simulink model "IEEE_14_Final"  (R2024a)
settings: Solver=FixedStepDiscrete  StartTime=0  StopTime=0.20000000000000001  FixedStep=0.00016666666666666666  RelTol=1e-4  AbsTol=1e-6  EnableMultiTasking=on
undefined symbols (not defined in the file or in its folder): D11, Delta
libraries: spsThreePhasePISectionLineLib x21, spsThreePhaseVIMeasurementLib x17, spsThreePhaseSeriesRLCLoadLib x11, spsGroundLib x9, spsThreePhaseTransformerTwoWindingsLib x6, spsThreePhaseFaultLib x4, spsSynchronousMachinepuStandardLib x3, spsThreePhaseParallelRLCBranchLib x3, sps_lib x1
settings Model: Creator=Bharath  LastModifiedBy=Shakkya Gamage
settings SolverCC: AutoScaleAbsTol=off  MaxConsecutiveMinStep=auto  ZeroCrossControl=DisableAll  AlgebraicLoopSolver=TrustRegion
settings DataIOCC: SaveFormat=Array  SignalLoggingSaveFormat=ModelDataLogs
settings OptimizationCC: ExpressionDepthLimit=2147483647  LifeSpan=inf
settings DebuggingCC: AlgebraicLoopMsg=none  UnderspecifiedInitializationDetection=Classic  MergeDetectMultiDrivingBlocksExec=none  FcnCallInpInsideContextMsg=warning  UnconnectedInputMsg=warning  UnconnectedLineMsg=warning  StateNameClashWarn=warning  SFUnexpectedBacktrackingDiag=warning  SFNoUnconditionalDefaultTransitionDiag=warning  SFExecutionAtInitializationDiag=none  ArithmeticOperatorsInVariantConditions=warning
settings HardwareCC: ProdBitPerPointer=32  ProdBitPerSizeT=32  ProdBitPerPtrDiffT=32  ProdLargestAtomicFloat=None  ProdIntDivRoundTo=Undefined  ProdEndianess=Unspecified  ProdWordSize=32  ProdHWDeviceType=32-bit Generic
settings ModelReferenceCC: PropagateSignalLabelsOutOfModel=off
settings SFSimCC: SimUseLocalCustomCode=off  CustomCodeUndefinedFunction=UseInterfaceOnly
settings RTWCC: RTWUseLocalCustomCode=off  GPUComputeCapability=3.5
settings CodeAppCC: StateflowObjectComments=on
settings GRTTargetCC: TargetLangStandard=C89/C90 (ANSI)  CombineOutputUpdateFcns=off  GRTInterface=on
settings ConfigComp: CovMetricSettings=dw  CovSaveCumulativeToWorkspaceVar=on  CovSaveSingleToWorkspaceVar=on  CovExternalEMLEnable=off
settings SimscapeCC: SimscapeNormalizeSystem=off

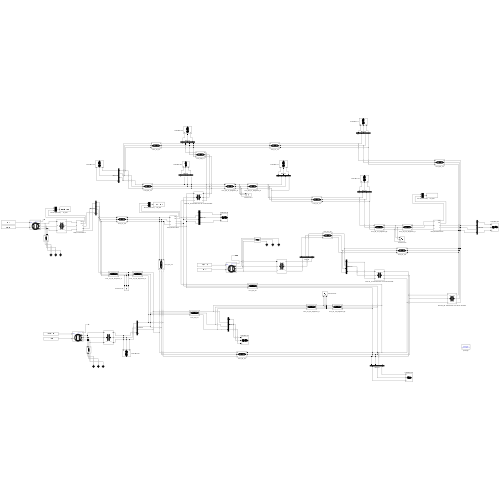
[thumbnail: Simulink's stored preview of the top-level diagram]
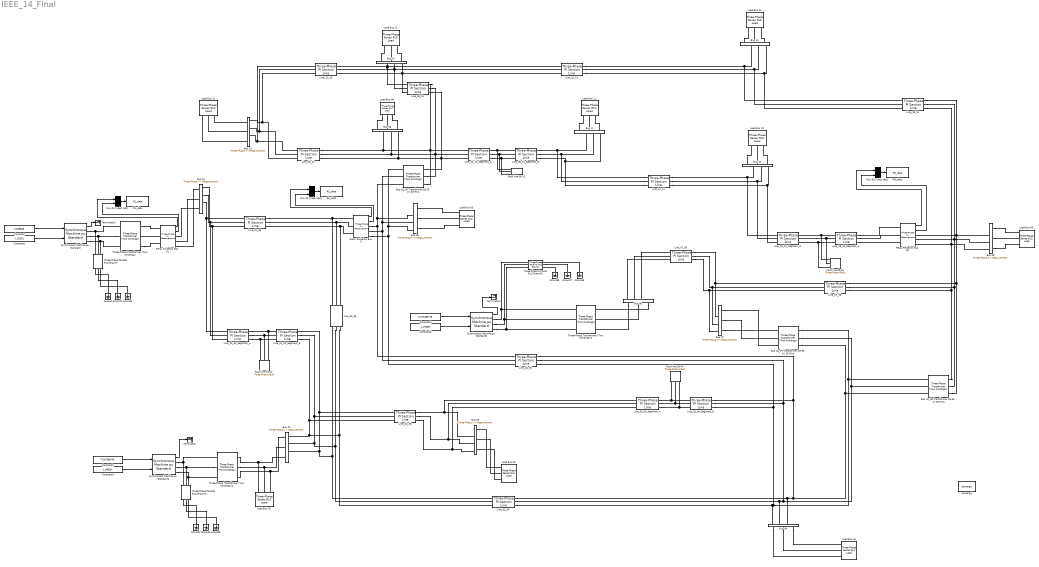
== system IEEE_14_Final ==
  Bus 01 : spsThreePhaseVIMeasurementLib/Three-Phase V-I Measurement  VoltageMeasurement=phase-to-ground  SetLabelV=off  LabelV=Vabc  Vpu=off  VpuLL=off  CurrentMeasurement=no  SetLabelI=off  LabelI=Iabc  Ipu=off  Pbase=31500000  Vbase=33000  OutputType=Complex  PhasorSimulation=off  PSBequivalent=0
  Bus 02 : spsThreePhaseVIMeasurementLib/Three-Phase V-I Measurement  VoltageMeasurement=phase-to-ground  SetLabelV=off  LabelV=Vabc  Vpu=off  VpuLL=off  CurrentMeasurement=no  SetLabelI=off  LabelI=Iabc  Ipu=off  Pbase=31500000  Vbase=33000  OutputType=Complex  PhasorSimulation=off  PSBequivalent=0
  Bus 03 : spsThreePhaseVIMeasurementLib/Three-Phase V-I Measurement  VoltageMeasurement=phase-to-ground  SetLabelV=off  LabelV=Vabc  Vpu=off  VpuLL=off  CurrentMeasurement=no  SetLabelI=off  LabelI=Iabc  Ipu=off  Pbase=31500000  Vbase=33000  OutputType=Complex  PhasorSimulation=off  PSBequivalent=0
  Bus 04 : spsThreePhaseVIMeasurementLib/Three-Phase V-I Measurement  VoltageMeasurement=phase-to-ground  SetLabelV=off  LabelV=Vabc  Vpu=off  VpuLL=off  CurrentMeasurement=no  SetLabelI=off  LabelI=Iabc  Ipu=off  Pbase=31500000  Vbase=33000  OutputType=Complex  PhasorSimulation=off  PSBequivalent=0
  Bus 04_07 Transformer 33-33 kV 50 MVA : spsThreePhaseTransformerTwoWindingsLib/Three-Phase Transformer (Two Windings)  Winding1Connection=Yg  Winding2Connection=Yg  CoreType=Three single-phase transformers  SetSaturation=off  Hysteresis=off  DataFile='hysteresis'  SetInitialFlux=off  Measurements=None  UNITS=pu  NominalPower=[50000000, 50]  Winding1=[33000 0.005 0.05]  Winding2=[33000 0.005 0.05]  Rm=500  Lm=500  L0=0.5  Saturation=[ 0,0 ; 0.0024,1.2 ; 1.0,1.52 ]  InitialFluxes=[ 0.8 , -0.8 , 0.7 ]  BreakLoop=off  DiscreteSolver=Trapezoidal iterative  DataType=off  TransfoNumber=1
  Bus 04_09 Transformer 33-33 kV 50 MVA : spsThreePhaseTransformerTwoWindingsLib/Three-Phase Transformer (Two Windings)  Winding1Connection=Yg  Winding2Connection=Yg  CoreType=Three single-phase transformers  SetSaturation=off  Hysteresis=off  DataFile='hysteresis'  SetInitialFlux=off  Measurements=None  UNITS=pu  NominalPower=[50000000, 50]  Winding1=[33000 0.005 0.14]  Winding2=[33000 0.005 0.14]  Rm=500  Lm=500  L0=0.5  Saturation=[ 0,0 ; 0.0024,1.2 ; 1.0,1.52 ]  InitialFluxes=[ 0.8 , -0.8 , 0.7 ]  BreakLoop=off  DiscreteSolver=Trapezoidal iterative  DataType=off  TransfoNumber=1
  Bus 05 : spsThreePhaseVIMeasurementLib/Three-Phase V-I Measurement  VoltageMeasurement=phase-to-ground  SetLabelV=off  LabelV=Vabc  Vpu=off  VpuLL=off  CurrentMeasurement=no  SetLabelI=off  LabelI=Iabc  Ipu=off  Pbase=31500000  Vbase=33000  OutputType=Complex  PhasorSimulation=off  PSBequivalent=0
  Bus 05_06 Transformer 33-33 kV 50 MVA : spsThreePhaseTransformerTwoWindingsLib/Three-Phase Transformer (Two Windings)  Winding1Connection=Yg  Winding2Connection=Yg  CoreType=Three single-phase transformers  SetSaturation=off  Hysteresis=off  DataFile='hysteresis'  SetInitialFlux=off  Measurements=None  UNITS=pu  NominalPower=[50000000, 50]  Winding1=[33000 0.005 0.063]  Winding2=[33000 0.005 0.063]  Rm=500  Lm=500  L0=0.5  Saturation=[ 0,0 ; 0.0024,1.2 ; 1.0,1.52 ]  InitialFluxes=[ 0.8 , -0.8 , 0.7 ]  BreakLoop=off  DiscreteSolver=Trapezoidal iterative  DataType=off  TransfoNumber=1
  Bus 06 : spsThreePhaseVIMeasurementLib/Three-Phase V-I Measurement  VoltageMeasurement=phase-to-ground  SetLabelV=off  LabelV=Vabc  Vpu=off  VpuLL=off  CurrentMeasurement=no  SetLabelI=off  LabelI=Iabc  Ipu=off  Pbase=31500000  Vbase=33000  OutputType=Complex  PhasorSimulation=off  PSBequivalent=0
  Bus 07 : spsThreePhaseVIMeasurementLib/Three-Phase V-I Measurement  VoltageMeasurement=phase-to-ground  SetLabelV=off  LabelV=Vabc  Vpu=off  VpuLL=off  CurrentMeasurement=no  SetLabelI=off  LabelI=Iabc  Ipu=off  Pbase=31500000  Vbase=33000  OutputType=Complex  PhasorSimulation=off  PSBequivalent=0
  Bus 08 : spsThreePhaseVIMeasurementLib/Three-Phase V-I Measurement  VoltageMeasurement=phase-to-ground  SetLabelV=off  LabelV=Vabc  Vpu=off  VpuLL=off  CurrentMeasurement=no  SetLabelI=off  LabelI=Iabc  Ipu=off  Pbase=31500000  Vbase=33000  OutputType=Complex  PhasorSimulation=off  PSBequivalent=0
  Bus 09 : spsThreePhaseVIMeasurementLib/Three-Phase V-I Measurement  VoltageMeasurement=phase-to-ground  SetLabelV=off  LabelV=Vabc  Vpu=off  VpuLL=off  CurrentMeasurement=no  SetLabelI=off  LabelI=Iabc  Ipu=off  Pbase=31500000  Vbase=33000  OutputType=Complex  PhasorSimulation=off  PSBequivalent=0
  Bus {10..14} (5 alike) : spsThreePhaseVIMeasurementLib/Three-Phase V-I Measurement  VoltageMeasurement=phase-to-ground  SetLabelV=off  LabelV=Vabc  Vpu=off  VpuLL=off  CurrentMeasurement=no  SetLabelI=off  LabelI=Iabc  Ipu=off  Pbase=31500000  Vbase=33000  OutputType=Complex  PhasorSimulation=off  PSBequivalent=0
  Constant : Constant  Value=0.205826
  Constant1 : Constant  Value=1.02301
  Constant2 : Constant  Value=7.51429e-06
  Constant3 : Constant  Value=1.09059
  Constant4 : Constant  Value=5.27348e-06
  Constant5 : Constant  Value=1.07589
  Fault line 01-02 : spsThreePhaseFaultLib/Three-Phase Fault  InitialStates=0  FaultA=off  FaultB=off  FaultC=off  GroundFault=off  SwitchTimes=[100 100.1]  External=off  SwitchStatus=NaN  FaultResistance=0.01  GroundResistance=0.001  SnubberResistance=1e6  SnubberCapacitance=inf  Measurements=None
  Fault line 03-04 : spsThreePhaseFaultLib/Three-Phase Fault  InitialStates=0  FaultA=off  FaultB=off  FaultC=off  GroundFault=off  SwitchTimes=[100 100.1]  External=off  SwitchStatus=NaN  FaultResistance=0.01  GroundResistance=0.001  SnubberResistance=1e6  SnubberCapacitance=inf  Measurements=None
  Fault line 06-11 : spsThreePhaseFaultLib/Three-Phase Fault  InitialStates=0  FaultA=off  FaultB=off  FaultC=off  GroundFault=off  SwitchTimes=[100 100.1]  External=off  SwitchStatus=NaN  FaultResistance=0.01  GroundResistance=0.001  SnubberResistance=1e6  SnubberCapacitance=inf  Measurements=None
  Fault line 09-10 : spsThreePhaseFaultLib/Three-Phase Fault  InitialStates=0  FaultA=on  FaultB=on  FaultC=on  GroundFault=off  SwitchTimes=[0.089158 0.128934]  External=off  SwitchStatus=NaN  FaultResistance=0.01  GroundResistance=0.001  SnubberResistance=1e6  SnubberCapacitance=inf  Measurements=None
  Ground{,1..8} (9 alike) : spsGroundLib/Ground  LConnTagsString=a
  Line_01_02_Segment_A : spsThreePhasePISectionLineLib/Three-Phase PI Section Line  LConnTagsString=A|B|C  RConnTagsString=A|B|C  Length=10  Frequency=50  Resistances=[0.16 0.48]  Inductances=[0.0012 0.0036]  Capacitances=[1e-08 6e-09]
  Line_01_02_Segment_B : spsThreePhasePISectionLineLib/Three-Phase PI Section Line  LConnTagsString=A|B|C  RConnTagsString=A|B|C  Length=10  Frequency=50  Resistances=[0.16 0.48]  Inductances=[0.0012 0.0036]  Capacitances=[1e-08 6e-09]
  Line_01_05 : spsThreePhasePISectionLineLib/Three-Phase PI Section Line  LConnTagsString=A|B|C  RConnTagsString=A|B|C  Length=15  Frequency=50  Resistances=[0.16 0.48]  Inductances=[0.0012 0.0036]  Capacitances=[1e-08 6e-09]
  Line_02_03 : spsThreePhasePISectionLineLib/Three-Phase PI Section Line  LConnTagsString=A|B|C  RConnTagsString=A|B|C  Length=12  Frequency=50  Resistances=[0.16 0.48]  Inductances=[0.0012 0.0036]  Capacitances=[1e-08 6e-09]
  Line_02_04 : spsThreePhasePISectionLineLib/Three-Phase PI Section Line  LConnTagsString=A|B|C  RConnTagsString=A|B|C  Length=10  Frequency=50  Resistances=[0.16 0.48]  Inductances=[0.0012 0.0036]  Capacitances=[1e-08 6e-09]
  Line_02_05 : spsThreePhasePISectionLineLib/Three-Phase PI Section Line  LConnTagsString=A|B|C  RConnTagsString=A|B|C  Length=8  Frequency=50  Resistances=[0.16 0.48]  Inductances=[0.0012 0.0036]  Capacitances=[1e-08 6e-09]
  Line_03_04_Segment_A : spsThreePhasePISectionLineLib/Three-Phase PI Section Line  LConnTagsString=A|B|C  RConnTagsString=A|B|C  Length=9  Frequency=50  Resistances=[0.16 0.48]  Inductances=[0.0012 0.0036]  Capacitances=[1e-08 6e-09]
  Line_03_04_Segment_B : spsThreePhasePISectionLineLib/Three-Phase PI Section Line  LConnTagsString=A|B|C  RConnTagsString=A|B|C  Length=9  Frequency=50  Resistances=[0.16 0.48]  Inductances=[0.0012 0.0036]  Capacitances=[1e-08 6e-09]
  Line_04_05 : spsThreePhasePISectionLineLib/Three-Phase PI Section Line  LConnTagsString=A|B|C  RConnTagsString=A|B|C  Length=7  Frequency=50  Resistances=[0.16 0.48]  Inductances=[0.0012 0.0036]  Capacitances=[1e-08 6e-09]
  Line_06_11_Segment_A : spsThreePhasePISectionLineLib/Three-Phase PI Section Line  LConnTagsString=A|B|C  RConnTagsString=A|B|C  Length=4  Frequency=50  Resistances=[0.16 0.48]  Inductances=[0.0012 0.0036]  Capacitances=[1e-08 6e-09]
  Line_06_11_Segment_B : spsThreePhasePISectionLineLib/Three-Phase PI Section Line  LConnTagsString=A|B|C  RConnTagsString=A|B|C  Length=4  Frequency=50  Resistances=[0.16 0.48]  Inductances=[0.0012 0.0036]  Capacitances=[1e-08 6e-09]
  Line_06_12 : spsThreePhasePISectionLineLib/Three-Phase PI Section Line  LConnTagsString=A|B|C  RConnTagsString=A|B|C  Length=12  Frequency=50  Resistances=[0.16 0.48]  Inductances=[0.0012 0.0036]  Capacitances=[1e-08 6e-09]
  Line_06_13 : spsThreePhasePISectionLineLib/Three-Phase PI Section Line  LConnTagsString=A|B|C  RConnTagsString=A|B|C  Length=15  Frequency=50  Resistances=[0.16 0.48]  Inductances=[0.0012 0.0036]  Capacitances=[1e-08 6e-09]
  Line_07_08 : spsThreePhasePISectionLineLib/Three-Phase PI Section Line  LConnTagsString=A|B|C  RConnTagsString=A|B|C  Length=5  Frequency=50  Resistances=[0.16 0.48]  Inductances=[0.0012 0.0036]  Capacitances=[1e-08 6e-09]
  Line_07_09 : spsThreePhasePISectionLineLib/Three-Phase PI Section Line  LConnTagsString=A|B|C  RConnTagsString=A|B|C  Length=8  Frequency=50  Resistances=[0.16 0.48]  Inductances=[0.0012 0.0036]  Capacitances=[1e-08 6e-09]
  Line_09_10_Segment_A : spsThreePhasePISectionLineLib/Three-Phase PI Section Line  LConnTagsString=A|B|C  RConnTagsString=A|B|C  Length=1.6926369239615902  Frequency=50  Resistances=[0.16 0.48]  Inductances=[0.0012 0.0036]  Capacitances=[1e-08 6e-09]
  Line_09_10_Segment_B : spsThreePhasePISectionLineLib/Three-Phase PI Section Line  LConnTagsString=A|B|C  RConnTagsString=A|B|C  Length=8.3073630760384098  Frequency=50  Resistances=[0.16 0.48]  Inductances=[0.0012 0.0036]  Capacitances=[1e-08 6e-09]
  Line_09_14 : spsThreePhasePISectionLineLib/Three-Phase PI Section Line  LConnTagsString=A|B|C  RConnTagsString=A|B|C  Length=14  Frequency=50  Resistances=[0.16 0.48]  Inductances=[0.0012 0.0036]  Capacitances=[1e-08 6e-09]
  Line_10_11 : spsThreePhasePISectionLineLib/Three-Phase PI Section Line  LConnTagsString=A|B|C  RConnTagsString=A|B|C  Length=6  Frequency=50  Resistances=[0.16 0.48]  Inductances=[0.0012 0.0036]  Capacitances=[1e-08 6e-09]
  Line_12_13 : spsThreePhasePISectionLineLib/Three-Phase PI Section Line  LConnTagsString=A|B|C  RConnTagsString=A|B|C  Length=5  Frequency=50  Resistances=[0.16 0.48]  Inductances=[0.0012 0.0036]  Capacitances=[1e-08 6e-09]
  Line_13_14 : spsThreePhasePISectionLineLib/Three-Phase PI Section Line  LConnTagsString=A|B|C  RConnTagsString=A|B|C  Length=7  Frequency=50  Resistances=[0.16 0.48]  Inductances=[0.0012 0.0036]  Capacitances=[1e-08 6e-09]
  Load Bus 02 : spsThreePhaseSeriesRLCLoadLib/Three-Phase Series RLC Load  LConnTagsString=A|B|C  Configuration=Y (grounded)  NominalVoltage=33000  Vabc=[1e3 1e3 1e3]  Vabcp=[1e3 1e3 1e3]  NominalFrequency=50  UnbalancedPower=off  ActivePower=500000  InductivePower=100000  CapacitivePower=0  Pabc=[10e3 9e3 11e3]  QLabc=[100 90 110]  QCabc=[100 90 110]  Pabcp=[10e3 9e3 11e3]  QLabcp=[100 90 110]  QCabcp=[100 90 110]  Measurements=None  LoadType=constant PQ
  Load Bus 03 : spsThreePhaseSeriesRLCLoadLib/Three-Phase Series RLC Load  LConnTagsString=A|B|C  Configuration=Y (grounded)  NominalVoltage=33000  Vabc=[1e3 1e3 1e3]  Vabcp=[1e3 1e3 1e3]  NominalFrequency=50  UnbalancedPower=off  ActivePower=500000  InductivePower=100000  CapacitivePower=0  Pabc=[10e3 9e3 11e3]  QLabc=[100 90 110]  QCabc=[100 90 110]  Pabcp=[10e3 9e3 11e3]  QLabcp=[100 90 110]  QCabcp=[100 90 110]  Measurements=None  LoadType=constant PQ
  Load Bus 04 : spsThreePhaseSeriesRLCLoadLib/Three-Phase Series RLC Load  LConnTagsString=A|B|C  Configuration=Y (grounded)  NominalVoltage=33000  Vabc=[1e3 1e3 1e3]  Vabcp=[1e3 1e3 1e3]  NominalFrequency=50  UnbalancedPower=off  ActivePower=3000000  InductivePower=0  CapacitivePower=0  Pabc=[10e3 9e3 11e3]  QLabc=[100 90 110]  QCabc=[100 90 110]  Pabcp=[10e3 9e3 11e3]  QLabcp=[100 90 110]  QCabcp=[100 90 110]  Measurements=None  LoadType=constant PQ
  Load Bus 05 : spsThreePhaseSeriesRLCLoadLib/Three-Phase Series RLC Load  LConnTagsString=A|B|C  Configuration=Y (grounded)  NominalVoltage=33000  Vabc=[1e3 1e3 1e3]  Vabcp=[1e3 1e3 1e3]  NominalFrequency=50  UnbalancedPower=off  ActivePower=500000  InductivePower=100000  CapacitivePower=0  Pabc=[10e3 9e3 11e3]  QLabc=[100 90 110]  QCabc=[100 90 110]  Pabcp=[10e3 9e3 11e3]  QLabcp=[100 90 110]  QCabcp=[100 90 110]  Measurements=None  LoadType=constant PQ
  Load Bus 06 : spsThreePhaseSeriesRLCLoadLib/Three-Phase Series RLC Load  LConnTagsString=A|B|C  Configuration=Y (grounded)  NominalVoltage=33000  Vabc=[1e3 1e3 1e3]  Vabcp=[1e3 1e3 1e3]  NominalFrequency=50  UnbalancedPower=off  ActivePower=500000  InductivePower=100000  CapacitivePower=0  Pabc=[10e3 9e3 11e3]  QLabc=[100 90 110]  QCabc=[100 90 110]  Pabcp=[10e3 9e3 11e3]  QLabcp=[100 90 110]  QCabcp=[100 90 110]  Measurements=None  LoadType=constant PQ
  Load Bus 09 : spsThreePhaseSeriesRLCLoadLib/Three-Phase Series RLC Load  LConnTagsString=A|B|C  Configuration=Y (grounded)  NominalVoltage=33000  Vabc=[1e3 1e3 1e3]  Vabcp=[1e3 1e3 1e3]  NominalFrequency=50  UnbalancedPower=off  ActivePower=1800000  InductivePower=1000000  CapacitivePower=0  Pabc=[10e3 9e3 11e3]  QLabc=[100 90 110]  QCabc=[100 90 110]  Pabcp=[10e3 9e3 11e3]  QLabcp=[100 90 110]  QCabcp=[100 90 110]  Measurements=None  LoadType=constant PQ
  Load Bus 10 : spsThreePhaseSeriesRLCLoadLib/Three-Phase Series RLC Load  LConnTagsString=A|B|C  Configuration=Y (grounded)  NominalVoltage=33000  Vabc=[1e3 1e3 1e3]  Vabcp=[1e3 1e3 1e3]  NominalFrequency=50  UnbalancedPower=off  ActivePower=600000  InductivePower=400000  CapacitivePower=0  Pabc=[10e3 9e3 11e3]  QLabc=[100 90 110]  QCabc=[100 90 110]  Pabcp=[10e3 9e3 11e3]  QLabcp=[100 90 110]  QCabcp=[100 90 110]  Measurements=None  LoadType=constant PQ
  Load Bus 11 : spsThreePhaseSeriesRLCLoadLib/Three-Phase Series RLC Load  LConnTagsString=A|B|C  Configuration=Y (grounded)  NominalVoltage=33000  Vabc=[1e3 1e3 1e3]  Vabcp=[1e3 1e3 1e3]  NominalFrequency=50  UnbalancedPower=off  ActivePower=200000  InductivePower=100000  CapacitivePower=0  Pabc=[10e3 9e3 11e3]  QLabc=[100 90 110]  QCabc=[100 90 110]  Pabcp=[10e3 9e3 11e3]  QLabcp=[100 90 110]  QCabcp=[100 90 110]  Measurements=None  LoadType=constant PQ
  Load Bus 12 : spsThreePhaseSeriesRLCLoadLib/Three-Phase Series RLC Load  LConnTagsString=A|B|C  Configuration=Y (grounded)  NominalVoltage=33000  Vabc=[1e3 1e3 1e3]  Vabcp=[1e3 1e3 1e3]  NominalFrequency=50  UnbalancedPower=off  ActivePower=400000  InductivePower=100000  CapacitivePower=0  Pabc=[10e3 9e3 11e3]  QLabc=[100 90 110]  QCabc=[100 90 110]  Pabcp=[10e3 9e3 11e3]  QLabcp=[100 90 110]  QCabcp=[100 90 110]  Measurements=None  LoadType=constant PQ
  Load Bus 13 : spsThreePhaseSeriesRLCLoadLib/Three-Phase Series RLC Load  LConnTagsString=A|B|C  Configuration=Y (grounded)  NominalVoltage=33000  Vabc=[1e3 1e3 1e3]  Vabcp=[1e3 1e3 1e3]  NominalFrequency=50  UnbalancedPower=off  ActivePower=800000  InductivePower=400000  CapacitivePower=0  Pabc=[10e3 9e3 11e3]  QLabc=[100 90 110]  QCabc=[100 90 110]  Pabcp=[10e3 9e3 11e3]  QLabcp=[100 90 110]  QCabcp=[100 90 110]  Measurements=None  LoadType=constant PQ
  Load Bus 14 : spsThreePhaseSeriesRLCLoadLib/Three-Phase Series RLC Load  LConnTagsString=A|B|C  Configuration=Y (grounded)  NominalVoltage=33000  Vabc=[1e3 1e3 1e3]  Vabcp=[1e3 1e3 1e3]  NominalFrequency=50  UnbalancedPower=off  ActivePower=900000  InductivePower=300000  CapacitivePower=0  Pabc=[10e3 9e3 11e3]  QLabc=[100 90 110]  QCabc=[100 90 110]  Pabcp=[10e3 9e3 11e3]  QLabcp=[100 90 110]  QCabcp=[100 90 110]  Measurements=None  LoadType=constant PQ
  Mux R1 [Vabc Iabc] : Mux  Inputs=2
  Mux R5 [Vabc Iabc] : Mux  Inputs=2
  Mux R9 [Vabc Iabc] : Mux  Inputs=2
  R1_data : ToWorkspace  VariableName=R1_data  SampleTime=-1
  R5_data : ToWorkspace  VariableName=R5_data  SampleTime=-1
  R9_data : ToWorkspace  VariableName=R9_data  SampleTime=-1
  Relay R1 below Bus 01 : spsThreePhaseVIMeasurementLib/Three-Phase V-I Measurement  VoltageMeasurement=phase-to-ground  SetLabelV=off  LabelV=Vabc  Vpu=off  VpuLL=off  CurrentMeasurement=yes  SetLabelI=off  LabelI=Iabc  Ipu=off  Pbase=31500000  Vbase=33000  OutputType=Complex  PhasorSimulation=off  PSBequivalent=0
  Relay R5 below Bus 5 : spsThreePhaseVIMeasurementLib/Three-Phase V-I Measurement  VoltageMeasurement=phase-to-ground  SetLabelV=off  LabelV=Vabc  Vpu=off  VpuLL=off  CurrentMeasurement=yes  SetLabelI=off  LabelI=Iabc  Ipu=off  Pbase=31500000  Vbase=33000  OutputType=Complex  PhasorSimulation=off  PSBequivalent=0
  Relay R9 below Bus 09 : spsThreePhaseVIMeasurementLib/Three-Phase V-I Measurement  VoltageMeasurement=phase-to-ground  SetLabelV=off  LabelV=Vabc  Vpu=off  VpuLL=off  CurrentMeasurement=yes  SetLabelI=off  LabelI=Iabc  Ipu=off  Pbase=31500000  Vbase=33000  OutputType=Complex  PhasorSimulation=off  PSBequivalent=0
  Synchronous Machine pu Standard : spsSynchronousMachinepuStandardLib/Synchronous Machine pu Standard  PresetModel=No  MechanicalLoad=Mechanical power Pm  ShowDetailedParameters=on  RotorType=Round  Units=per unit standard parameters  MeasurementBus=off  NominalParameters=[50e6 11e3 50]  Reactances1=[1.81 0.30 0.23 1.76 0.65 0.25 0.15]  Reactances2=[2.24 0.17 0.12 1.02 0.13 0.08]  dAxisTimeConstants=Open-circuit  qAxisTimeConstants=Open-circuit  TimeConstants1="[ 4.4849  0.0681  0.1  ]"  TimeConstants2=[ 8.0, 0.03, 1.0, 0.07 ]  TimeConstants3="[  4.49  0.0681  0.0513  ]"  TimeConstants4=[ 8.0, 0.03, 0.3371, 0.0295 ]  TimeConstants5=[ 1.01, 0.053, 0.1 ]  TimeConstants6=[ 1.3201, 0.023, 1.0, 0.07 ]  TimeConstants7=[0.012 0.003 0.003]  TimeConstants8=[ 8.0 0.03 1.0 0.07 ]  StatorResistance=0.003  Mechanical=[3.5 0 1]  PolePairs=20  InitialConditions=[0 -69.219 0.20738 0.20738 0.20738 7.30633 -112.694 127.306 1.02301]  SetSaturation=off  Saturation=[0.6404,0.7127,0.8441,0.9214,0.9956,1.082,1.19,1.316,1.457;0.7,0.7698,0.8872,0.9466,0.9969,1.046,1.1,1.151,1.201]  LoadFlowParameters=[2 0 0 0 0]  TsPowergui=0  TsBlock=-1  IterativeModel=Trapezoidal non iterative  IterativeDiscreteModel=Trapezoidal robust  BusType=swing  Pref=0  Qref=0  Qmin=-inf  Qmax=inf  PLF=0  QLF=0
  Synchronous Machine pu Standard1 : spsSynchronousMachinepuStandardLib/Synchronous Machine pu Standard  PresetModel=No  MechanicalLoad=Mechanical power Pm  ShowDetailedParameters=on  RotorType=Round  Units=per unit standard parameters  MeasurementBus=off  NominalParameters=[50e6 11e3 50]  Reactances1=[1.81 0.30 0.23 1.76 0.65 0.25 0.15]  Reactances2=[2.24 0.17 0.12 1.02 0.13 0.08]  dAxisTimeConstants=Open-circuit  qAxisTimeConstants=Open-circuit  TimeConstants1="[ 4.4849  0.0681  0.1  ]"  TimeConstants2=[ 8.0, 0.03, 1.0, 0.07 ]  TimeConstants3="[  4.49  0.0681  0.0513  ]"  TimeConstants4=[ 8.0, 0.03, 0.3371, 0.0295 ]  TimeConstants5=[ 1.01, 0.053, 0.1 ]  TimeConstants6=[ 1.3201, 0.023, 1.0, 0.07 ]  TimeConstants7=[0.012 0.003 0.003]  TimeConstants8=[ 8.0 0.03 1.0 0.07 ]  StatorResistance=0.003  Mechanical=[3.5 0 1]  PolePairs=20  InitialConditions=[0 -93.0795 0.0500476 0.0500476 0.0500476 -93.0716 146.928 26.9284 1.09059]  SetSaturation=off  Saturation=[0.6404,0.7127,0.8441,0.9214,0.9956,1.082,1.19,1.316,1.457;0.7,0.7698,0.8872,0.9466,0.9969,1.046,1.1,1.151,1.201]  LoadFlowParameters=[1 0 0 0 0]  TsPowergui=0  TsBlock=-1  IterativeModel=Trapezoidal non iterative  IterativeDiscreteModel=Trapezoidal robust  BusType=swing  Pref=0  Qref=0  Qmin=-inf  Qmax=inf  PLF=0  QLF=0
  Synchronous Machine pu Standard2 : spsSynchronousMachinepuStandardLib/Synchronous Machine pu Standard  PresetModel=No  MechanicalLoad=Mechanical power Pm  ShowDetailedParameters=on  RotorType=Round  Units=per unit standard parameters  MeasurementBus=off  NominalParameters=[50e6 11e3 50]  Reactances1=[1.81 0.30 0.23 1.76 0.65 0.25 0.15]  Reactances2=[2.24 0.17 0.12 1.02 0.13 0.08]  dAxisTimeConstants=Open-circuit  qAxisTimeConstants=Open-circuit  TimeConstants1="[ 4.4849  0.0681  0.1  ]"  TimeConstants2=[ 8.0, 0.03, 1.0, 0.07 ]  TimeConstants3="[  4.49  0.0681  0.0513  ]"  TimeConstants4=[ 8.0, 0.03, 0.3371, 0.0295 ]  TimeConstants5=[ 1.01, 0.053, 0.1 ]  TimeConstants6=[ 1.3201, 0.023, 1.0, 0.07 ]  TimeConstants7=[0.012 0.003 0.003]  TimeConstants8=[ 8.0 0.03 1.0 0.07 ]  StatorResistance=0.003  Mechanical=[3.5 0 1]  PolePairs=20  InitialConditions=[0 -93.7473 0.0419264 0.0419264 0.0419264 -93.7406 146.259 26.2594 1.07589]  SetSaturation=off  Saturation=[0.6404,0.7127,0.8441,0.9214,0.9956,1.082,1.19,1.316,1.457;0.7,0.7698,0.8872,0.9466,0.9969,1.046,1.1,1.151,1.201]  LoadFlowParameters=[1 0 0 0 0]  TsPowergui=0  TsBlock=-1  IterativeModel=Trapezoidal non iterative  IterativeDiscreteModel=Trapezoidal robust  BusType=swing  Pref=0  Qref=0  Qmin=-inf  Qmax=inf  PLF=0  QLF=0
  Terminator : Terminator
  Terminator1 : Terminator
  Terminator2 : Terminator
  Three-Phase Parallel RLC Branch : spsThreePhaseParallelRLCBranchLib/Three-Phase Parallel RLC Branch  LConnTagsString=A|B|C  RConnTagsString=A|B|C  BranchType=R  Resistance=1e6  Inductance=1e-3  Capacitance=1e-6  Measurements=None
  Three-Phase Parallel RLC Branch1 : spsThreePhaseParallelRLCBranchLib/Three-Phase Parallel RLC Branch  LConnTagsString=A|B|C  RConnTagsString=A|B|C  BranchType=R  Resistance=1e6  Inductance=1e-3  Capacitance=1e-6  Measurements=None
  Three-Phase Parallel RLC Branch2 : spsThreePhaseParallelRLCBranchLib/Three-Phase Parallel RLC Branch  LConnTagsString=A|B|C  RConnTagsString=A|B|C  BranchType=R  Resistance=1e6  Inductance=1e-3  Capacitance=1e-6  Measurements=None
  Three-Phase Transformer (Two Windings) : spsThreePhaseTransformerTwoWindingsLib/Three-Phase Transformer (Two Windings)  Winding1Connection=Delta (D11)  Winding2Connection=Yg  CoreType=Three single-phase transformers  SetSaturation=off  Hysteresis=off  DataFile='hysteresis'  SetInitialFlux=off  Measurements=None  UNITS=pu  NominalPower=[ 50e6 , 50 ]  Winding1=[ 11e3 , 0.005 , 0.05 ]  Winding2=[ 33e3 , 0.005 , 0.05 ]  Rm=500  Lm=500  L0=0.5  Saturation=[ 0,0 ; 0.0024,1.2 ; 1.0,1.52 ]  InitialFluxes=[ 0.8 , -0.8 , 0.7 ]  BreakLoop=off  DiscreteSolver=Trapezoidal iterative  DataType=off  TransfoNumber=1
  Three-Phase Transformer (Two Windings)1 : spsThreePhaseTransformerTwoWindingsLib/Three-Phase Transformer (Two Windings)  Winding1Connection=Delta (D11)  Winding2Connection=Yg  CoreType=Three single-phase transformers  SetSaturation=off  Hysteresis=off  DataFile='hysteresis'  SetInitialFlux=off  Measurements=None  UNITS=pu  NominalPower=[ 50e6 , 50 ]  Winding1=[ 11e3 , 0.005 , 0.05 ]  Winding2=[ 33e3 , 0.005 , 0.05 ]  Rm=500  Lm=500  L0=0.5  Saturation=[ 0,0 ; 0.0024,1.2 ; 1.0,1.52 ]  InitialFluxes=[ 0.8 , -0.8 , 0.7 ]  BreakLoop=off  DiscreteSolver=Trapezoidal iterative  DataType=off  TransfoNumber=1
  Three-Phase Transformer (Two Windings)2 : spsThreePhaseTransformerTwoWindingsLib/Three-Phase Transformer (Two Windings)  Winding1Connection=Delta (D11)  Winding2Connection=Yg  CoreType=Three single-phase transformers  SetSaturation=off  Hysteresis=off  DataFile='hysteresis'  SetInitialFlux=off  Measurements=None  UNITS=pu  NominalPower=[ 50e6 , 50 ]  Winding1=[ 11e3 , 0.005 , 0.05 ]  Winding2=[ 33e3 , 0.005 , 0.05 ]  Rm=500  Lm=500  L0=0.5  Saturation=[ 0,0 ; 0.0024,1.2 ; 1.0,1.52 ]  InitialFluxes=[ 0.8 , -0.8 , 0.7 ]  BreakLoop=off  DiscreteSolver=Trapezoidal iterative  DataType=off  TransfoNumber=1
  powergui : sps_lib/powergui  Priority=1  SimulationMode=Discrete  SampleTime=1/6000  frequency=50  Iterations=50  frequencyindice=50  Pbase=31500000  ErrMax=1e-4  UnitsV=kV  UnitsW=MW  buscounter=0  FunctionMessages=off  echomessages=off  EnableUseOfTLC=off  CurrentSourceSwitches=on  DisableSnubberDevices=off  DisableRonSwitches=off  DisableVfSwitches=off  DisplayEquations=off  AutomaticDiscreteSolvers=off  SolverType=Tustin  Interpol=off  ExternalGateDelay=off  methode=off  Ts=100  x0status=blocks  SPID=off  SwTol=0  HookPort=off  NonlinearTolerance=1e-4  nMaxIteration=100  ContinueOnMaxIteration=off  RestoreLinks=warning  ResistiveCurrentMeasurement=off  Frange=[0:2:500]  Ylog=off  Xlog=on  ShowGrid=off  save=off  variable=ZData  structure=0  ZoomFFT=off  StartTime=0.0  cycles=1  DisplayStyle=1  fundamental=50  FreqAxis=off  MaxFrequency=3000  frequencyindicesteady=1  RmsSteady=1  display=off
  wires:
  Relay R1 below Bus 01/1 -> Mux R1 [Vabc Iabc]/1
  Relay R1 below Bus 01/2 -> Mux R1 [Vabc Iabc]/2
  Mux R1 [Vabc Iabc]/1 -> R1_data/1
  Mux R9 [Vabc Iabc]/1 -> R9_data/1
  Relay R9 below Bus 09/2 -> Mux R9 [Vabc Iabc]/2
  Relay R9 below Bus 09/1 -> Mux R9 [Vabc Iabc]/1
  Mux R5 [Vabc Iabc]/1 -> R5_data/1
  Relay R5 below Bus 5/2 -> Mux R5 [Vabc Iabc]/2
  Relay R5 below Bus 5/1 -> Mux R5 [Vabc Iabc]/1
  Constant1/1 -> Synchronous Machine pu Standard/2
  Constant/1 -> Synchronous Machine pu Standard/1
  Constant2/1 -> Synchronous Machine pu Standard1/1
  Constant3/1 -> Synchronous Machine pu Standard1/2
  Constant4/1 -> Synchronous Machine pu Standard2/1
  Constant5/1 -> Synchronous Machine pu Standard2/2
  Synchronous Machine pu Standard1/1 -> Terminator/1
  Synchronous Machine pu Standard/1 -> Terminator1/1
  Synchronous Machine pu Standard2/1 -> Terminator2/1
  connections:
  Bus 01/RConn1 -- Line_01_02_Segment_A/LConn1 -- Line_01_05/LConn1
  Line_01_05/RConn1 -- Relay R5 below Bus 5/LConn1 -- Line_02_05/RConn1
  Bus 08/RConn1 -- Line_07_08/RConn1
  Bus 01/RConn2 -- Line_01_05/LConn2 -- Line_01_02_Segment_A/LConn2
  Line_04_05/LConn2 -- Relay R5 below Bus 5/RConn2 -- Bus 05/RConn2 -- Bus 05_06 Transformer 33-33 kV 50 MVA/LConn2
  Bus 08/RConn2 -- Line_07_08/RConn2
  Bus 01/RConn3 -- Line_01_02_Segment_A/LConn3 -- Line_01_05/LConn3
  Line_04_05/LConn3 -- Relay R5 below Bus 5/RConn3 -- Bus 05/RConn3 -- Bus 05_06 Transformer 33-33 kV 50 MVA/LConn3
  Bus 08/RConn3 -- Line_07_08/RConn3
  Load Bus 03/LConn1 -- Bus 03/LConn1
  Load Bus 03/LConn2 -- Bus 03/LConn2
  Load Bus 03/LConn3 -- Bus 03/LConn3
  Bus 04/LConn1 -- Load Bus 04/LConn1
  Bus 04/LConn2 -- Load Bus 04/LConn2
  Bus 04/LConn3 -- Load Bus 04/LConn3
  Bus 05/LConn1 -- Load Bus 05/LConn1
  Bus 05/LConn2 -- Load Bus 05/LConn2
  Bus 05/LConn3 -- Load Bus 05/LConn3
  Load Bus 06/LConn1 -- Bus 06/LConn1
  Load Bus 06/LConn2 -- Bus 06/LConn2
  Load Bus 06/LConn3 -- Bus 06/LConn3
  Bus 09/LConn1 -- Load Bus 09/LConn1
  Bus 09/LConn2 -- Load Bus 09/LConn2
  Bus 09/LConn3 -- Load Bus 09/LConn3
  Bus 10/LConn1 -- Load Bus 10/LConn1
  Bus 10/LConn2 -- Load Bus 10/LConn2
  Bus 10/LConn3 -- Load Bus 10/LConn3
  Bus 11/LConn1 -- Load Bus 11/LConn1
  Bus 11/LConn2 -- Load Bus 11/LConn2
  Bus 11/LConn3 -- Load Bus 11/LConn3
  Bus 12/LConn1 -- Load Bus 12/LConn1
  Bus 12/LConn2 -- Load Bus 12/LConn2
  Bus 12/LConn3 -- Load Bus 12/LConn3
  Bus 13/LConn1 -- Load Bus 13/LConn1
  Bus 13/LConn2 -- Load Bus 13/LConn2
  Bus 13/LConn3 -- Load Bus 13/LConn3
  Bus 14/LConn1 -- Load Bus 14/LConn1
  Bus 14/LConn2 -- Load Bus 14/LConn2
  Bus 14/LConn3 -- Load Bus 14/LConn3
  Relay R1 below Bus 01/RConn1 -- Bus 01/LConn1
  Relay R1 below Bus 01/RConn2 -- Bus 01/LConn2
  Relay R1 below Bus 01/RConn3 -- Bus 01/LConn3
  Line_01_02_Segment_A/RConn1 -- Line_01_02_Segment_B/LConn1 -- Fault line 01-02/LConn1
  Line_01_02_Segment_A/RConn2 -- Fault line 01-02/LConn2 -- Line_01_02_Segment_B/LConn2
  Line_01_02_Segment_A/RConn3 -- Line_01_02_Segment_B/LConn3 -- Fault line 01-02/LConn3
  Line_03_04_Segment_A/RConn1 -- Line_03_04_Segment_B/LConn1 -- Fault line 03-04/LConn1
  Line_03_04_Segment_A/RConn2 -- Line_03_04_Segment_B/LConn2 -- Fault line 03-04/LConn2
  Line_03_04_Segment_A/RConn3 -- Line_03_04_Segment_B/LConn3 -- Fault line 03-04/LConn3
  Line_09_10_Segment_A/RConn1 -- Fault line 09-10/LConn1 -- Line_09_10_Segment_B/LConn1
  Line_09_10_Segment_A/RConn2 -- Fault line 09-10/LConn2 -- Line_09_10_Segment_B/LConn2
  Line_09_10_Segment_A/RConn3 -- Fault line 09-10/LConn3 -- Line_09_10_Segment_B/LConn3
  Line_01_02_Segment_B/RConn1 -- Line_02_04/LConn1 -- Line_02_05/LConn1 -- Bus 02/RConn1 -- Line_02_03/LConn1
  Line_01_02_Segment_B/RConn2 -- Line_02_05/LConn2 -- Line_02_04/LConn2 -- Bus 02/RConn2 -- Line_02_03/LConn2
  Line_01_02_Segment_B/RConn3 -- Line_02_04/LConn3 -- Line_02_05/LConn3 -- Bus 02/RConn3 -- Line_02_03/LConn3
  Line_02_03/RConn1 -- Line_03_04_Segment_A/LConn1 -- Bus 03/RConn1
  Line_02_03/RConn2 -- Line_03_04_Segment_A/LConn2 -- Bus 03/RConn2
  Line_02_03/RConn3 -- Line_03_04_Segment_A/LConn3 -- Bus 03/RConn3
  Line_06_13/LConn1 -- Bus 05_06 Transformer 33-33 kV 50 MVA/RConn1 -- Line_06_11_Segment_A/RConn1 -- Line_06_12/LConn1 -- Bus 06/RConn1
  Line_06_12/LConn2 -- Bus 06/RConn2 -- Bus 05_06 Transformer 33-33 kV 50 MVA/RConn2 -- Line_06_11_Segment_A/RConn2 -- Line_06_13/LConn2
  Line_06_11_Segment_A/RConn3 -- Bus 05_06 Transformer 33-33 kV 50 MVA/RConn3 -- Line_06_13/LConn3 -- Line_06_12/LConn3 -- Bus 06/RConn3
  Line_06_12/RConn3 -- Line_12_13/RConn3 -- Bus 12/RConn3
  Line_06_12/RConn2 -- Line_12_13/RConn2 -- Bus 12/RConn2
  Line_06_12/RConn1 -- Line_12_13/RConn1 -- Bus 12/RConn1
  Line_10_11/LConn1 -- Bus 11/RConn1 -- Line_06_11_Segment_B/LConn1
  Line_10_11/LConn2 -- Bus 11/RConn2 -- Line_06_11_Segment_B/LConn2
  Line_10_11/LConn3 -- Bus 11/RConn3 -- Line_06_11_Segment_B/LConn3
  Line_12_13/LConn1 -- Bus 13/RConn1 -- Line_06_13/RConn1 -- Line_13_14/RConn1
  Bus 13/RConn2 -- Line_12_13/LConn2 -- Line_06_13/RConn2 -- Line_13_14/RConn2
  Bus 13/RConn3 -- Line_12_13/LConn3 -- Line_06_13/RConn3 -- Line_13_14/RConn3
  Line_13_14/LConn1 -- Bus 14/RConn1 -- Line_09_14/RConn1
  Line_13_14/LConn2 -- Line_09_14/RConn2 -- Bus 14/RConn2
  Line_13_14/LConn3 -- Line_09_14/RConn3 -- Bus 14/RConn3
  Line_10_11/RConn1 -- Line_09_10_Segment_B/RConn1 -- Bus 10/RConn1
  Line_10_11/RConn2 -- Bus 10/RConn2 -- Line_09_10_Segment_B/RConn2
  Line_10_11/RConn3 -- Line_09_10_Segment_B/RConn3 -- Bus 10/RConn3
  Bus 09/RConn3 -- Line_07_09/LConn3 -- Bus 04_09 Transformer 33-33 kV 50 MVA/RConn3 -- Relay R9 below Bus 09/RConn3 -- Line_09_14/LConn3
  Bus 09/RConn2 -- Line_09_14/LConn2 -- Bus 04_09 Transformer 33-33 kV 50 MVA/RConn2 -- Line_07_09/LConn2 -- Relay R9 below Bus 09/RConn2
  Bus 09/RConn1 -- Bus 04_09 Transformer 33-33 kV 50 MVA/RConn1 -- Line_07_09/LConn1 -- Relay R9 below Bus 09/RConn1 -- Line_09_14/LConn1
  Line_02_04/RConn1 -- Bus 04/RConn1 -- Bus 04_07 Transformer 33-33 kV 50 MVA/RConn1 -- Bus 04_09 Transformer 33-33 kV 50 MVA/LConn1 -- Line_04_05/RConn1 -- Line_03_04_Segment_B/RConn1
  Line_02_04/RConn2 -- Bus 04/RConn2 -- Bus 04_07 Transformer 33-33 kV 50 MVA/RConn2 -- Bus 04_09 Transformer 33-33 kV 50 MVA/LConn2 -- Line_04_05/RConn2 -- Line_03_04_Segment_B/RConn2
  Line_02_04/RConn3 -- Bus 04/RConn3 -- Bus 04_07 Transformer 33-33 kV 50 MVA/RConn3 -- Bus 04_09 Transformer 33-33 kV 50 MVA/LConn3 -- Line_04_05/RConn3 -- Line_03_04_Segment_B/RConn3
  Line_07_09/RConn1 -- Line_07_08/LConn1 -- Bus 07/RConn1
  Line_07_09/RConn2 -- Line_07_08/LConn2 -- Bus 07/RConn2
  Line_07_09/RConn3 -- Line_07_08/LConn3 -- Bus 07/RConn3
  Line_09_10_Segment_A/LConn1 -- Relay R9 below Bus 09/LConn1
  Line_09_10_Segment_A/LConn2 -- Relay R9 below Bus 09/LConn2
  Line_09_10_Segment_A/LConn3 -- Relay R9 below Bus 09/LConn3
  Load Bus 02/LConn2 -- Bus 02/LConn2 -- Three-Phase Transformer (Two Windings)1/RConn2
  Load Bus 02/LConn1 -- Bus 02/LConn1 -- Three-Phase Transformer (Two Windings)1/RConn1
  Load Bus 02/LConn3 -- Bus 02/LConn3 -- Three-Phase Transformer (Two Windings)1/RConn3
  Line_06_11_Segment_A/LConn1 -- Fault line 06-11/LConn1 -- Line_06_11_Segment_B/RConn1
  Line_06_11_Segment_A/LConn2 -- Fault line 06-11/LConn2 -- Line_06_11_Segment_B/RConn2
  Line_06_11_Segment_A/LConn3 -- Fault line 06-11/LConn3 -- Line_06_11_Segment_B/RConn3
  Bus 07/LConn2 -- Bus 04_07 Transformer 33-33 kV 50 MVA/LConn2
  Bus 07/LConn1 -- Bus 04_07 Transformer 33-33 kV 50 MVA/LConn1
  Bus 07/LConn3 -- Bus 04_07 Transformer 33-33 kV 50 MVA/LConn3
  Bus 05/RConn1 -- Relay R5 below Bus 5/RConn1 -- Line_04_05/LConn1 -- Bus 05_06 Transformer 33-33 kV 50 MVA/LConn1
  Line_01_05/RConn2 -- Relay R5 below Bus 5/LConn2 -- Line_02_05/RConn2
  Line_02_05/RConn3 -- Relay R5 below Bus 5/LConn3 -- Line_01_05/RConn3
  Three-Phase Parallel RLC Branch/LConn1 -- Synchronous Machine pu Standard/RConn1 -- Three-Phase Transformer (Two Windings)/LConn1
  Three-Phase Parallel RLC Branch/LConn3 -- Synchronous Machine pu Standard/RConn3 -- Three-Phase Transformer (Two Windings)/LConn3
  Three-Phase Transformer (Two Windings)/LConn2 -- Synchronous Machine pu Standard/RConn2 -- Three-Phase Parallel RLC Branch/LConn2
  Relay R1 below Bus 01/LConn2 -- Three-Phase Transformer (Two Windings)/RConn2
  Ground2/LConn1 -- Three-Phase Parallel RLC Branch/RConn3
  Three-Phase Transformer (Two Windings)/RConn3 -- Relay R1 below Bus 01/LConn3
  Ground/LConn1 -- Three-Phase Parallel RLC Branch/RConn1
  Three-Phase Transformer (Two Windings)/RConn1 -- Relay R1 below Bus 01/LConn1
  Three-Phase Parallel RLC Branch/RConn2 -- Ground1/LConn1
  Three-Phase Parallel RLC Branch1/LConn1 -- Synchronous Machine pu Standard1/RConn1 -- Three-Phase Transformer (Two Windings)1/LConn1
  Three-Phase Parallel RLC Branch1/LConn3 -- Synchronous Machine pu Standard1/RConn3 -- Three-Phase Transformer (Two Windings)1/LConn3
  Three-Phase Transformer (Two Windings)1/LConn2 -- Synchronous Machine pu Standard1/RConn2 -- Three-Phase Parallel RLC Branch1/LConn2
  Ground5/LConn1 -- Three-Phase Parallel RLC Branch1/RConn3
  Three-Phase Parallel RLC Branch1/RConn2 -- Ground4/LConn1
  Ground3/LConn1 -- Three-Phase Parallel RLC Branch1/RConn1
  Three-Phase Parallel RLC Branch2/LConn1 -- Synchronous Machine pu Standard2/RConn1 -- Three-Phase Transformer (Two Windings)2/LConn1
  Three-Phase Parallel RLC Branch2/LConn3 -- Synchronous Machine pu Standard2/RConn3 -- Three-Phase Transformer (Two Windings)2/LConn3
  Three-Phase Parallel RLC Branch2/LConn2 -- Synchronous Machine pu Standard2/RConn2 -- Three-Phase Transformer (Two Windings)2/LConn2
  Ground8/LConn1 -- Three-Phase Parallel RLC Branch2/RConn3
  Three-Phase Parallel RLC Branch2/RConn2 -- Ground7/LConn1
  Ground6/LConn1 -- Three-Phase Parallel RLC Branch2/RConn1
  Bus 08/LConn3 -- Three-Phase Transformer (Two Windings)2/RConn3
  Bus 08/LConn2 -- Three-Phase Transformer (Two Windings)2/RConn2
  Bus 08/LConn1 -- Three-Phase Transformer (Two Windings)2/RConn1
